simulink model "new_foc_mmd"  (R2024b)
settings: Solver=VariableStepAuto  StartTime=0.0  StopTime=3.14  FixedStep=0.000001  MaxStep=1e-4  RelTol=1e-3
model workspace (MAT data in the model file):
  fs = 4000
undefined symbols (not defined in the file): speed_ref, Ts
libraries: simulink x13, spsIGBTDiodeLib x6, slpidlib x3, spsVoltageMeasurementLib x3, spsPermanentMagnetSynchronousMachineLib x1, spsDCVoltageSourceLib x1, spsSawtoothGeneratorLib x1, simulink_extras x1, spsThreePhaseVIMeasurementLib x1, spspowerguiLib x1
(part 2 of 2)

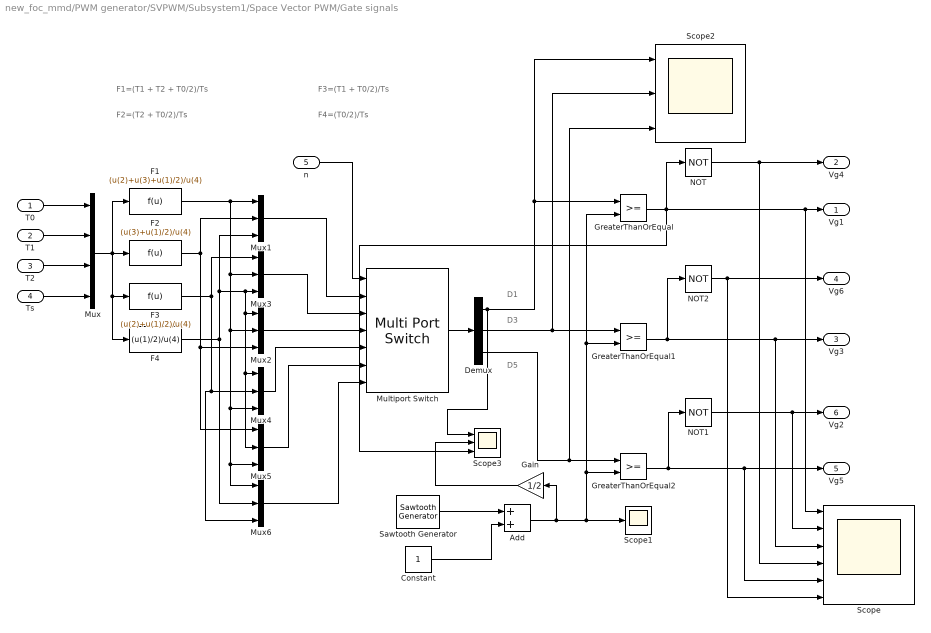
== system new_foc_mmd/PWM generator/SVPWM/Subsystem1/Space Vector PWM/Gate signals ==
  note: D1
  note: F1=(T1 + T2 + T0/2)/Ts
  note: F2=(T2 + T0/2)/Ts
  note: F3=(T1 + T0/2)/Ts
  note: F4=(T0/2)/Ts
  note: D3
  note: D5
  T0 : Inport
  T1 : Inport  Port=2
  T2 : Inport  Port=3
  Ts : Inport  Port=4
  n : Inport  Port=5
  Add : Sum
  Constant : Constant
  Demux : Demux  Outputs=3
  F1 : Fcn  Expr=(u(2)+u(3)+u(1)/2)/u(4)
  F2 : Fcn  Expr=(u(3)+u(1)/2)/u(4)
  F3 : Fcn  Expr=(u(2)+u(1)/2)/u(4)
  F4 : Fcn  Expr=(u(1)/2)/u(4)
  Gain : Gain  Gain=1/2
  GreaterThanOrEqual : RelationalOperator  OutDataTypeStr=boolean  RndMeth=Simplest  InputSameDT=off
  GreaterThanOrEqual1 : RelationalOperator  OutDataTypeStr=boolean  RndMeth=Simplest  InputSameDT=off
  GreaterThanOrEqual2 : RelationalOperator  OutDataTypeStr=boolean  RndMeth=Simplest  InputSameDT=off
  Multiport Switch : MultiPortSwitch  Inputs=6  DiagnosticForDefault=None  SaturateOnIntegerOverflow=off  InputSameDT=off
  Mux : Mux
  Mux{1..6} (6 alike) : Mux  Inputs=3
  NOT : Logic  Operator=NOT  IconShape=distinctive  AllPortsSameDT=off  OutDataTypeStr=boolean
  NOT1 : Logic  Operator=NOT  IconShape=distinctive  AllPortsSameDT=off  OutDataTypeStr=boolean
  NOT2 : Logic  Operator=NOT  IconShape=distinctive  AllPortsSameDT=off  OutDataTypeStr=boolean
  Sawtooth Generator : spsSawtoothGeneratorLib/Sawtooth Generator  Freq=5e3  Phase=0  Ts=0
  Scope : Scope  NumInputPorts=6
  Scope1 : Scope
  Scope2 : Scope  NumInputPorts=3
  Scope3 : Scope  NumInputPorts=3
  Vg1 : Outport  VectorParamsAs1DForOutWhenUnconnected=off
  Vg4 : Outport  Port=2  VectorParamsAs1DForOutWhenUnconnected=off
  Vg3 : Outport  Port=3  VectorParamsAs1DForOutWhenUnconnected=off
  Vg6 : Outport  Port=4  VectorParamsAs1DForOutWhenUnconnected=off
  Vg5 : Outport  Port=5  VectorParamsAs1DForOutWhenUnconnected=off
  Vg2 : Outport  Port=6  VectorParamsAs1DForOutWhenUnconnected=off
  wires:
  Demux/2 -> GreaterThanOrEqual1/1, Scope2/2
  Sawtooth Generator/1 -> Add/1
  GreaterThanOrEqual/1 -> Scope3/3, Scope/1, Vg1/1, NOT/1
  GreaterThanOrEqual1/1 -> NOT2/1, Scope/3, Vg3/1
  GreaterThanOrEqual2/1 -> NOT1/1, Scope/5, Vg5/1
  NOT/1 -> Scope/4, Vg4/1
  NOT1/1 -> Scope/2, Vg2/1
  NOT2/1 -> Scope/6, Vg6/1
  n/1 -> Multiport Switch/1
  T0/1 -> Mux/1
  T1/1 -> Mux/2
  T2/1 -> Mux/3
  Ts/1 -> Mux/4
  Mux/1 -> F1/1, F2/1, F4/1, F3/1
  Demux/3 -> GreaterThanOrEqual2/1, Scope2/3
  Add/1 -> Gain/1, Scope1/1, GreaterThanOrEqual2/2, GreaterThanOrEqual1/2, GreaterThanOrEqual/2
  Constant/1 -> Add/2
  Multiport Switch/1 -> Demux/1
  Demux/1 -> Scope3/1, GreaterThanOrEqual/1, Scope2/1
  Mux6/1 -> Multiport Switch/7
  Mux5/1 -> Multiport Switch/6
  Mux4/1 -> Multiport Switch/5
  Mux2/1 -> Multiport Switch/4
  Mux3/1 -> Multiport Switch/3
  Mux1/1 -> Multiport Switch/2
  F1/1 -> Mux6/1, Mux5/3, Mux4/3, Mux2/2, Mux3/2, Mux1/1
  F2/1 -> Mux1/2, Mux5/1, Mux2/3
  F4/1 -> Mux6/2, Mux5/2, Mux4/1, Mux2/1, Mux3/3, Mux1/3
  F3/1 -> Mux6/3, Mux4/2, Mux3/1
  Gain/1 -> Scope3/2

== system new_foc_mmd/PWM generator/SVPWM/Subsystem1/Space Vector PWM/Modulation index ==
  Vref : Inport
  Abs : Abs  SaturateOnIntegerOverflow=off
  Fcn1 : Fcn  Expr=u(1)/((2/3)*u(2))
  M1 : Constant  Value=0.86
  Mux : Mux  Inputs=2
  Scope : Scope
  Switch : Switch  Threshold=0.866  SaturateOnIntegerOverflow=off  InputSameDT=off
  Vs : Constant  Value=106.67
  a : Outport  VectorParamsAs1DForOutWhenUnconnected=off
  wires:
  Fcn1/1 -> Switch/3, Switch/2
  Vs/1 -> Mux/2
  M1/1 -> Switch/1
  Vref/1 -> Abs/1
  Mux/1 -> Fcn1/1
  Switch/1 -> Scope/1, a/1
  Abs/1 -> Mux/1

== system new_foc_mmd/PWM generator/SVPWM/Subsystem1/Space Vector PWM/T0_T1_T2 ==
  alpha : Inport
  n : Inport  Port=2
  a : Inport  Port=3
  Ts : Inport  Port=4
  Mux : Mux
  Scope1 : Scope  NumInputPorts=3
  Sum : Sum  Inputs=|--+
  T_1 : Fcn  Expr=(u(3)*u(4)*(sin((u(2)*pi/3)-u(1)*pi/180)))/(sin(pi/3))
  T_2 : Fcn  Expr=(u(3)*u(4)*(sin(u(1)*pi/180-((u(2)-1)*pi/3))))/(sin(pi/3))
  T0 : Outport  VectorParamsAs1DForOutWhenUnconnected=off
  T1 : Outport  Port=2  VectorParamsAs1DForOutWhenUnconnected=off
  T2 : Outport  Port=3  VectorParamsAs1DForOutWhenUnconnected=off
  wires:
  Mux/1 -> T_2/1, T_1/1
  n/1 -> Mux/2
  a/1 -> Mux/3
  Ts/1 -> Sum/3, Mux/4
  T_2/1 -> Sum/2, Scope1/3, T2/1
  T_1/1 -> Scope1/1, T1/1, Sum/1
  Sum/1 -> Scope1/2, T0/1
  alpha/1 -> Mux/1

== system new_foc_mmd/PWM generator/SVPWM/Subsystem1/Space Vector PWM/Vref and angle calclator ==
  Valpha : Inport
  Vbeta : Inport  Port=2
  Complex to Magnitude-Angle : ComplexToMagnitudeAngle
  Real-Imag to Complex : RealImagToComplex
  rad to deg : Subsystem
  alpha : Outport  VectorParamsAs1DForOutWhenUnconnected=off
  Vref : Outport  Port=2  VectorParamsAs1DForOutWhenUnconnected=off
  wires:
  Valpha/1 -> Real-Imag to Complex/1
  Real-Imag to Complex/1 -> Complex to Magnitude-Angle/1
  Vbeta/1 -> Real-Imag to Complex/2
  rad to deg/1(2D) -> alpha/1
  Complex to Magnitude-Angle/2 -> rad to deg/1(R)
  Complex to Magnitude-Angle/1 -> Vref/1

== system new_foc_mmd/PWM generator/SVPWM/Subsystem1/Space Vector PWM/Vref and angle calclator/rad to deg ==
  R : Inport
  Constant1 : Constant  Value=2*pi
  Radians to Degrees1 : simulink_extras/Transformations/Radians to Degrees
  Sum : Sum  Inputs=|++
  Switch : Switch  SaturateOnIntegerOverflow=off  InputSameDT=off
  2D : Outport  VectorParamsAs1DForOutWhenUnconnected=off
  wires:
  R/1 -> Switch/2, Switch/1, Sum/1
  Radians to Degrees1/1 -> 2D/1
  Switch/1 -> Radians to Degrees1/1
  Sum/1 -> Switch/3
  Constant1/1 -> Sum/2
